simulink model "sldemo_VariableTransportDelay_pipe"  (R2023b)
settings: Solver=ode45  StartTime=0.0  StopTime=10.0  MaxStep=0.01  RelTol=1e-3  EnableMultiTasking=on
libraries: simulink x2
Description:
  | Incompressible flow through a fixed length pipe
  | 
  | An incompressible flow goes through a pipe of length L with speed v(t).
  | At the inlet the flow temperature is Ti, then the temperature at the
  | outletTo can be modeled as an variable transport delay of  Ti. At time
  | t=0, the pipe is empty and  until t=2, there is no flow at the outlet.
  | Thus the output temperature before t=2 is the initial output temperature.
settings Model: Creator=The MathWorks, Inc.  LastModifiedBy=The MathWorks, Inc.
settings SolverCC: AlgebraicLoopSolver=TrustRegion
settings DataIOCC: LimitDataPoints=on  SaveFormat=Array
settings OptimizationCC: ExpressionDepthLimit=2147483647  InitFltsAndDblsToZero=on  LifeSpan=inf
settings DebuggingCC: SaveWithParameterizedLinksMsg=none  UnderspecifiedInitializationDetection=Classic  MergeDetectMultiDrivingBlocksExec=none  SignalResolutionControl=TryResolveAllWithWarning  SolverPrmCheckMsg=warning  MultiTaskDSMMsg=warning  MultiTaskCondExecSysMsg=none  FcnCallInpInsideContextMsg=warning  UnconnectedInputMsg=warning  UnconnectedOutputMsg=warning  UnconnectedLineMsg=warning  StateNameClashWarn=warning  SFUnexpectedBacktrackingDiag=warning  SFNoUnconditionalDefaultTransitionDiag=warning  SFExecutionAtInitializationDiag=none  ArithmeticOperatorsInVariantConditions=warning
settings HardwareCC: ProdBitPerPointer=32  ProdBitPerSizeT=32  ProdBitPerPtrDiffT=32  ProdLargestAtomicFloat=None  ProdIntDivRoundTo=Undefined  ProdEndianess=Unspecified  ProdWordSize=32  ProdHWDeviceType=32-bit Generic
settings ModelReferenceCC: EnableRefExpFcnMdlSchedulingChecks=on  PropagateSignalLabelsOutOfModel=off
settings SFSimCC: SimUseLocalCustomCode=off  CustomCodeUndefinedFunction=UseInterfaceOnly
settings RTWCC: RTWUseLocalCustomCode=off
settings CodeAppCC: StateflowObjectComments=on
settings GRTTargetCC: TargetFcnLib=ansi_tfl_tmw.mat  TargetLangStandard=C89/C90 (ANSI)  CombineOutputUpdateFcns=off  GRTInterface=on
settings ConfigComp: CovMetricSettings=dw  CovSaveCumulativeToWorkspaceVar=on  CovSaveSingleToWorkspaceVar=on  CovExternalEMLEnable=off

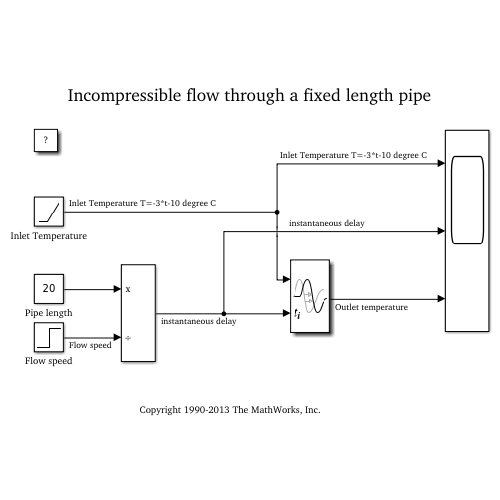
[thumbnail: Simulink's stored preview of the top-level diagram]
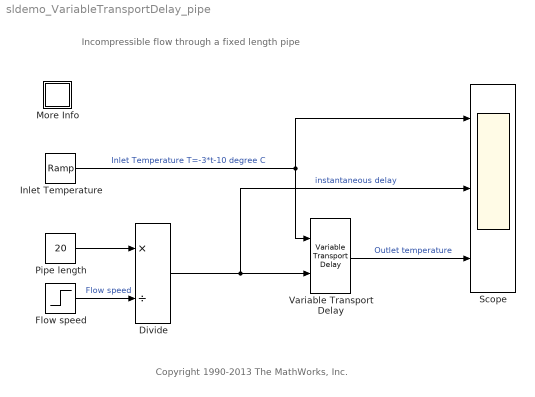
== system sldemo_VariableTransportDelay_pipe ==
  note: Incompressible flow through a fixed length pipe
  note: Copyright 1990-2013 The MathWorks, Inc.
  Divide : Product  Inputs=*/
  Flow speed : Step  Time=5  Before=10  After=20  SampleTime=0
  Inlet Temperature : simulink/Sources/Ramp  slope=3  start=0  InitialOutput=-10
  More Info : Subsystem
      settings: OpenFcn=showExample('simulink_general/sldemo_VariableTransportDelayExample')
      mask Display: disp('?')
  Pipe length : Constant  Value=20
  Scope : Scope  NumInputPorts=3
  Variable Transport Delay : VariableTransportDelay  VariableDelayType=Variable transport delay  MaximumDelay=1000  InitialOutput=-15
  wires:
  Variable Transport Delay/1 -> Scope/3  "Outlet temperature"
  Divide/1 -> Scope/2, Variable Transport Delay/2  "instantaneous delay"
  Flow speed/1 -> Divide/2  "Flow speed"
  Pipe length/1 -> Divide/1
  Inlet Temperature/1 -> Scope/1, Variable Transport Delay/1  "Inlet Temperature T=-3*t-10 degree C"

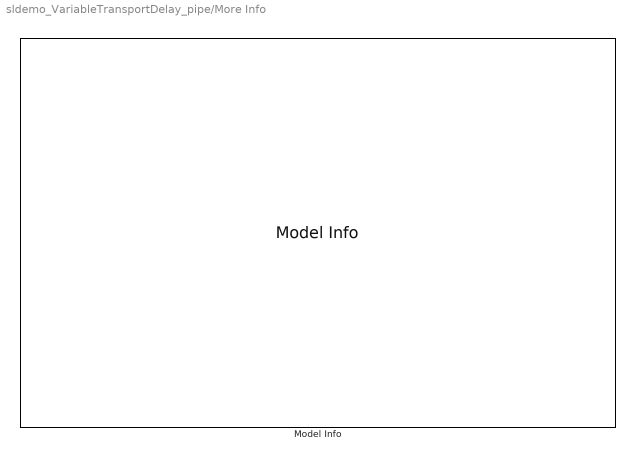
== system sldemo_VariableTransportDelay_pipe/More Info ==
  Model Info : simulink/Model-Wide Utilities/Model Info  Frame=on  DisplayStringWithTags=Model Info  HorizontalTextAlignment=Left  LeftAlignmentValue=0.02
